simulink model "AA2"  (R2021a)
settings: Solver=VariableStepAuto  StartTime=0.0  StopTime=10  RelTol=1e-3
libraries: simulink x1, ctrlSharedLib x1
settings Model: Creator=jhaid  LastModifiedBy=jhaid

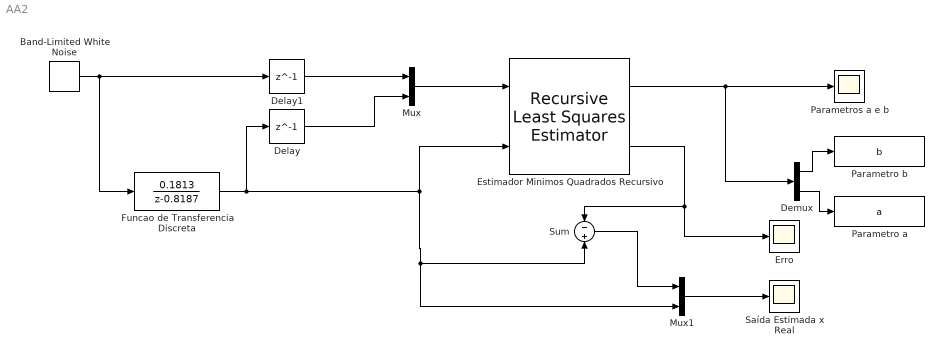
== system AA2 ==
  Band-Limited White Noise : simulink/Sources/Band-Limited White Noise  Cov=[0.1]  Ts=0.1  seed=[23341]
  Delay : Delay  DelayLength=1  InitialCondition=0
  Delay1 : Delay  DelayLength=1  InitialCondition=0
  Demux : Demux  Outputs=2
  Erro : Scope
  Estimador Minimos Quadrados Recursivo : ctrlSharedLib/Recursive Least Squares Estimator  InitialEstimateSource=Internal  InitialParameterData=[1 1]  P0=1e4  InitialRegressors=0  InitialOutputs=0  History=Infinite  WindowLength=200  EstimationMethod=Forgetting Factor  AdaptationParameter=1  HasTimeVaryingAdaptationParameter=off  NormalizationBias=eps  OutputError=on  OutputP=off  AddEnablePort=off  InputProcessing=Sample-based  Ts=-1
      settings: SourceProductBaseCode=CT,ID
  Funcao de Transferencia Discreta : DiscreteTransferFcn  Numerator=0.1813  Denominator="[1   -0.8187]"
  Mux : Mux  Inputs=2
  Mux1 : Mux  Inputs=2
  Parametro a : ToWorkspace  VariableName=a  SampleTime=-1
  Parametro b : ToWorkspace  VariableName=b  SampleTime=-1
  Parametros a e b : Scope
  Saída Estimada x Real : Scope
  Sum : Sum  Inputs=-+
  wires:
  Delay/1 -> Mux/2
  Mux/1 -> Estimador Minimos Quadrados Recursivo/1
  Funcao de Transferencia Discreta/1 -> Delay/1, Estimador Minimos Quadrados Recursivo/2, Mux1/2, Sum/2
  Estimador Minimos Quadrados Recursivo/2 -> Erro/1, Sum/1
  Sum/1 -> Mux1/1
  Mux1/1 -> Saída Estimada x Real/1
  Estimador Minimos Quadrados Recursivo/1 -> Demux/1, Parametros a e b/1
  Band-Limited White Noise/1 -> Delay1/1, Funcao de Transferencia Discreta/1
  Demux/1 -> Parametro b/1
  Demux/2 -> Parametro a/1
  Delay1/1 -> Mux/1
